simulink model "Induction_electromagnetique"  (R2017b)
settings: Solver=VariableStepAuto  StartTime=0.0  StopTime=inf  FixedStep=1/5000  RelTol=1e-3
libraries: fl_lib x16, Library_SII x4, nesl_utility x4, peRmsMeasurement x2
settings Model: Creator=Cedrick  LastModifiedBy=Cedrick

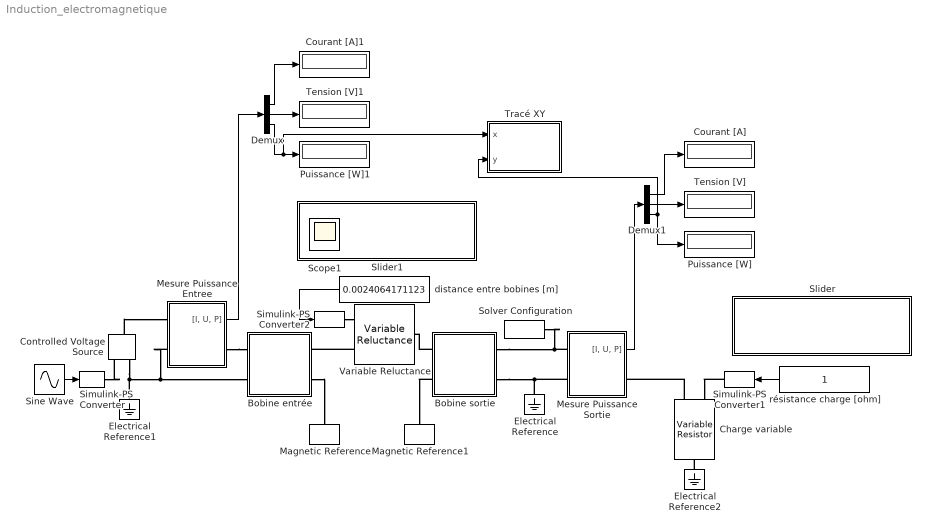
== system Induction_electromagnetique ==
  Bobine entrée : Subsystem  mask{N=30, s=1e-6, D=0.1, l=0.01}
      mask prompts: N "Nombre de tours"; s "Section du fil [m²]"; D "Diamètre de la bobine [m]"; l "Longueur de la bobine [m]"
      mask init:
      | % Perméabilité magnétique du vide
      | mu0 = pi*4e-7;
      | 
      | % Résistivité cuivre
      | rho = 1.7e-8; % Ohm.m
      mask DialogControl s Tooltip: Section du fil constituant la bobine
  Bobine sortie : Subsystem  mask{N=30, s=1e-6, D=0.1, l=0.01}
      mask prompts: N "Nombre de tours"; s "Section du fil [m²]"; D "Diamètre de la bobine [m]"; l "Longueur de la bobine [m]"
      mask init:
      | % Perméabilité magnétique du vide
      | mu0 = pi*4e-7;
      | 
      | % Résistivité cuivre
      | rho = 1.7e-8; % Ohm.m
      mask DialogControl s Tooltip: Section du fil constituant la bobine
  Charge variable : fl_lib/Electrical/Electrical Elements/Variable Resistor  Rmin=1 Ohm  i_specify=off  i_priority=None  i=0 A  i_nominal_specify=off  i_nominal_unit=A  i_nominal_value=1  v_specify=off  v_priority=None  v=0 V  v_nominal_specify=off  v_nominal_unit=V  v_nominal_value=1
  Controlled Voltage Source : fl_lib/Electrical/Electrical Sources/Controlled Voltage Source
  Courant [A] : Display
  Courant [A]1 : Display
  Demux : Demux  Outputs=3
  Demux1 : Demux  Outputs=3
  Electrical Reference : fl_lib/Electrical/Electrical Elements/Electrical Reference
  Electrical Reference1 : fl_lib/Electrical/Electrical Elements/Electrical Reference
  Electrical Reference2 : fl_lib/Electrical/Electrical Elements/Electrical Reference
  Magnetic Reference : fl_lib/Magnetic/Magnetic Elements/Magnetic Reference
      settings: SourceProductName=Simscape  SourceProductBaseCode=SS
  Magnetic Reference1 : fl_lib/Magnetic/Magnetic Elements/Magnetic Reference
      settings: SourceProductName=Simscape  SourceProductBaseCode=SS
  Mesure Puissance Entree : Subsystem  mask(Mesure de puissance Electrique RMS){ff=50}
      mask prompts: ff "Fréquence fondamentale [Hz]"
      mask help:
      | Mesure le courant, la tension et la puissance RMS sur un circuit.
      | Retourne les valeurs sous forme d'un vecteur [I, U, P]
      mask init:
      | fs = get_param(bdroot, 'FixedStep');
      | 
      | % Longueur de la fenêtre de mesure RMS
      | lw = int32(ff*fs)
      mask Display: disp('RMS')
  Mesure Puissance Sortie : Subsystem  mask(Mesure de puissance Electrique RMS){ff=50}
      mask prompts: ff "Fréquence fondamentale [Hz]"
      mask help:
      | Mesure le courant, la tension et la puissance RMS sur un circuit.
      | Retourne les valeurs sous forme d'un vecteur [I, U, P]
      mask init:
      | fs = get_param(bdroot, 'FixedStep');
      | 
      | % Longueur de la fenêtre de mesure RMS
      | lw = int32(ff*fs)
      mask Display: disp('RMS')
  Puissance [W] : Display
  Puissance [W]1 : Display
  Simulink-PS Converter : nesl_utility/Simulink-PS Converter  PhysicalDomain=network_engine_domain  SubClassName=ps_input  LeftPortType=input  RightPortType=output  PseudoPeriodic=off  Frequencies=[]  NoiseDistribution=none  NoiseParameters=[]  Unit=1  AffineConversion=off  FilteringAndDerivatives=provide  SimscapeFilterOrder=1  InputFilterTimeConstant=0.001  UdotUserProvided=0
  Simulink-PS Converter1 : nesl_utility/Simulink-PS Converter  PhysicalDomain=network_engine_domain  SubClassName=ps_input  LeftPortType=input  RightPortType=output  PseudoPeriodic=off  Frequencies=[]  NoiseDistribution=none  NoiseParameters=[]  Unit=1  AffineConversion=off  FilteringAndDerivatives=provide  SimscapeFilterOrder=1  InputFilterTimeConstant=0.001  UdotUserProvided=0
  Simulink-PS Converter2 : nesl_utility/Simulink-PS Converter  PhysicalDomain=network_engine_domain  SubClassName=ps_input  LeftPortType=input  RightPortType=output  PseudoPeriodic=off  Frequencies=[]  NoiseDistribution=none  NoiseParameters=[]  Unit=1  AffineConversion=off  FilteringAndDerivatives=provide  SimscapeFilterOrder=1  InputFilterTimeConstant=0.001  UdotUserProvided=0
  Sine Wave : Sin  Amplitude=5  Frequency=50*2*pi  SampleTime=0
  Slider : Subsystem  DialogController=hmiCreateDDGDialog  IsWebBlock=on  mask(MWDashboardBlock){webBlockId=574ab3c5-b9e4-429a-9142-107109e8eed0, webBlockType=slider, ShowInLibBrowser=on, ShowInitialText=on, HMISrcModelName=Induction}
      mask prompts: webBlockId "WebBlock Id"; webBlockType "WebBlock Type"; HMISrcModelName "Source Model"
      mask help: SimulinkHMI:dialogs:SliderDialogDesc
      mask Help: helpview([docroot '/mapfiles/simulink.map'], 'hmi_slider')
      mask Display:
      | if strcmp(get_param(bdroot(gcb),'BlockDiagramType'), 'library')
      |     image([(matlabroot) '/toolbox/simulink/hmi/icons/Slider.png']);
      | end
  Slider1 : Subsystem  DialogController=hmiCreateDDGDialog  IsWebBlock=on  mask(MWDashboardBlock){webBlockId=ceebdebb-3da2-42cb-9bc8-324251df0c3a, webBlockType=slider, ShowInLibBrowser=on, ShowInitialText=on, HMISrcModelName=Induction}
      mask prompts: webBlockId "WebBlock Id"; webBlockType "WebBlock Type"; HMISrcModelName "Source Model"
      mask help: SimulinkHMI:dialogs:SliderDialogDesc
      mask Help: helpview([docroot '/mapfiles/simulink.map'], 'hmi_slider')
      mask Display:
      | if strcmp(get_param(bdroot(gcb),'BlockDiagramType'), 'library')
      |     image([(matlabroot) '/toolbox/simulink/hmi/icons/Slider.png']);
      | end
  Solver Configuration : nesl_utility/Solver Configuration  PhysicalDomain=network_engine_domain  SubClassName=solver  LeftPortType=input  RightPortType=generic  Accelerate=off  Tones=[]  Harmonics=[]  SimulateNoise=off  Profile=off  UseLocalSampling=off  EnableSwitchedLinearOptims=on  FrequencyDomain=off  UseCCode=off  RelTol=0.001  AbsTol=1e-06  MinStep=1e-09  ToWorkspace=off  RevertToSquareIcSolve=off  NumHomotopyIterations=100  PhasorMode=off  PhasorModeNumHarmonics=1  DoDC=off  ResidualTolerance=1e-09  UseLocalSolver=off  LocalSolverChoice=NE_BACKWARD_EULER_ADVANCER  LocalSolverSampleTime=0.001  DoFixedCost=off  MaxNonlinIter=3  MaxModeIter=2  LinearAlgebra=Sparse  DelaysMemoryBudget=1024  AutomaticFiltering=on  FilteringTimeConstant=0.001
  Tension [V] : Display
  Tension [V]1 : Display
  Tracé XY : MATLAB Function  TreatAsAtomicUnit=on  SystemSampleTime=10
  Variable Reluctance : fl_lib/Magnetic/Magnetic Elements/Variable Reluctance  Xmin=0 m  CSA=pi*0.1^2/4 m^2  mur=1  phi_specify=off  phi_priority=None  phi=0 Wb  phi_nominal_specify=off  phi_nominal_unit=Wb  phi_nominal_value=1  mmf_specify=off  mmf_priority=None  mmf=0 A  mmf_nominal_specify=off  mmf_nominal_unit=A  mmf_nominal_value=1
      settings: SourceProductName=Simscape  SourceProductBaseCode=SS
  distance entre bobines [m] : Constant  Value=0.0024064171123
  résistance charge [ohm] : Constant
  Scope1 : Scope
  wires:
  Sine Wave/1 -> Simulink-PS Converter/1
  résistance charge [ohm]/1 -> Simulink-PS Converter1/1
  Demux1/1 -> Courant [A]/1
  Demux1/2 -> Tension [V]/1
  Demux1/3 -> Puissance [W]/1, Tracé XY/2(y)
  Demux/1 -> Courant [A]1/1
  Demux/2 -> Tension [V]1/1
  distance entre bobines [m]/1 -> Simulink-PS Converter2/1
  Demux/3 -> Tracé XY/1(x), Puissance [W]1/1
  Mesure Puissance Entree/1("[I, U, P]") -> Demux/1
  Mesure Puissance Sortie/1("[I, U, P]") -> Demux1/1
  connections:
  Bobine sortie/RConn1 -- Variable Reluctance/RConn1
  Solver Configuration/RConn1 -- Bobine sortie/LConn1 -- Mesure Puissance Sortie/LConn1
  Electrical Reference/LConn1 -- Bobine sortie/LConn2 -- Mesure Puissance Sortie/LConn2
  Controlled Voltage Source/RConn2 -- Electrical Reference1/LConn1 -- Mesure Puissance Entree/LConn2 -- Bobine entrée/LConn2
  Simulink-PS Converter/RConn1 -- Controlled Voltage Source/RConn1
  Variable Reluctance/LConn1 -- Bobine entrée/RConn1
  Simulink-PS Converter1/RConn1 -- Charge variable/LConn1
  Charge variable/LConn2 -- Mesure Puissance Sortie/RConn1
  Electrical Reference2/LConn1 -- Charge variable/RConn1
  Controlled Voltage Source/LConn1 -- Mesure Puissance Entree/LConn1
  Bobine sortie/RConn2 -- Magnetic Reference1/LConn1
  Bobine entrée/RConn2 -- Magnetic Reference/LConn1
  Mesure Puissance Entree/RConn1 -- Bobine entrée/LConn1
  Simulink-PS Converter2/RConn1 -- Variable Reluctance/LConn2

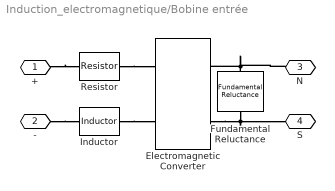
== system Induction_electromagnetique/Bobine entrée ==
  Electromagnetic Converter : fl_lib/Magnetic/Magnetic Elements/Electromagnetic Converter  Nw=N  i_specify=off  i_priority=None  i=0 A  i_nominal_specify=off  i_nominal_unit=A  i_nominal_value=1  v_specify=off  v_priority=None  v=0 V  v_nominal_specify=off  v_nominal_unit=V  v_nominal_value=1  mmf_specify=off  mmf_priority=None  mmf=0 A  mmf_nominal_specify=off  mmf_nominal_unit=A  mmf_nominal_value=1  phi_specify=off  phi_priority=High  phi=0 Wb  phi_nominal_specify=off  phi_nominal_unit=Wb  phi_nominal_value=1
      settings: SourceProductName=Simscape  SourceProductBaseCode=SS
  Fundamental Reluctance : fl_lib/Magnetic/Magnetic Elements/Fundamental Reluctance  R=4*l/(mu0*pi*D^2) 1/H  phi_specify=off  phi_priority=None  phi=0 Wb  phi_nominal_specify=off  phi_nominal_unit=Wb  phi_nominal_value=1  mmf_specify=off  mmf_priority=None  mmf=0 A  mmf_nominal_specify=off  mmf_nominal_unit=A  mmf_nominal_value=1
      settings: SourceProductName=Simscape  SourceProductBaseCode=SS
  Inductor : fl_lib/Electrical/Electrical Elements/Inductor  l=mu0*pi*D^2/4*N^2/l H  r=0 Ohm  g=1e-20 1/Ohm  i_specify=off  i_priority=None  i=0 A  i_nominal_specify=off  i_nominal_unit=A  i_nominal_value=1  v_specify=off  v_priority=None  v=0 V  v_nominal_specify=off  v_nominal_unit=V  v_nominal_value=1  i_L_specify=off  i_L_priority=High  i_L=0 A  i_L_nominal_specify=off  i_L_nominal_unit=A  i_L_nominal_value=1
  Resistor : fl_lib/Electrical/Electrical Elements/Resistor  R=rho*pi*D*N/s Ohm  i_specify=off  i_priority=None  i=0 A  i_nominal_specify=off  i_nominal_unit=A  i_nominal_value=1  v_specify=off  v_priority=None  v=0 V  v_nominal_specify=off  v_nominal_unit=V  v_nominal_value=1
  + : PMIOPort  Port=1  Side=Left
  - : PMIOPort  Port=2  Side=Left
  N : PMIOPort  Port=3  Side=Right
  S : PMIOPort  Port=4  Side=Right
  connections:
  Fundamental Reluctance/LConn1 -- Electromagnetic Converter/RConn1 -- N/RConn1
  Resistor/RConn1 -- Electromagnetic Converter/LConn1
  Electromagnetic Converter/RConn2 -- Fundamental Reluctance/RConn1 -- S/RConn1
  Inductor/RConn1 -- Electromagnetic Converter/LConn2
  +/RConn1 -- Resistor/LConn1
  -/RConn1 -- Inductor/LConn1

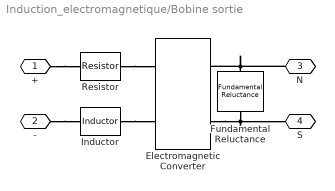
== system Induction_electromagnetique/Bobine sortie ==
  Electromagnetic Converter : fl_lib/Magnetic/Magnetic Elements/Electromagnetic Converter  Nw=N  i_specify=off  i_priority=None  i=0 A  i_nominal_specify=off  i_nominal_unit=A  i_nominal_value=1  v_specify=off  v_priority=None  v=0 V  v_nominal_specify=off  v_nominal_unit=V  v_nominal_value=1  mmf_specify=off  mmf_priority=None  mmf=0 A  mmf_nominal_specify=off  mmf_nominal_unit=A  mmf_nominal_value=1  phi_specify=off  phi_priority=High  phi=0 Wb  phi_nominal_specify=off  phi_nominal_unit=Wb  phi_nominal_value=1
      settings: SourceProductName=Simscape  SourceProductBaseCode=SS
  Fundamental Reluctance : fl_lib/Magnetic/Magnetic Elements/Fundamental Reluctance  R=4*l/(mu0*pi*D^2) 1/H  phi_specify=off  phi_priority=None  phi=0 Wb  phi_nominal_specify=off  phi_nominal_unit=Wb  phi_nominal_value=1  mmf_specify=off  mmf_priority=None  mmf=0 A  mmf_nominal_specify=off  mmf_nominal_unit=A  mmf_nominal_value=1
      settings: SourceProductName=Simscape  SourceProductBaseCode=SS
  Inductor : fl_lib/Electrical/Electrical Elements/Inductor  l=mu0*pi*D^2/4*N^2/l H  r=0 Ohm  g=1e-20 1/Ohm  i_specify=off  i_priority=None  i=0 A  i_nominal_specify=off  i_nominal_unit=A  i_nominal_value=1  v_specify=off  v_priority=None  v=0 V  v_nominal_specify=off  v_nominal_unit=V  v_nominal_value=1  i_L_specify=off  i_L_priority=High  i_L=0 A  i_L_nominal_specify=off  i_L_nominal_unit=A  i_L_nominal_value=1
  Resistor : fl_lib/Electrical/Electrical Elements/Resistor  R=rho*pi*D*N/s Ohm  i_specify=off  i_priority=None  i=0 A  i_nominal_specify=off  i_nominal_unit=A  i_nominal_value=1  v_specify=off  v_priority=None  v=0 V  v_nominal_specify=off  v_nominal_unit=V  v_nominal_value=1
  + : PMIOPort  Port=1  Side=Left
  - : PMIOPort  Port=2  Side=Left
  N : PMIOPort  Port=3  Side=Right
  S : PMIOPort  Port=4  Side=Right
  connections:
  N/RConn1 -- Fundamental Reluctance/LConn1 -- Electromagnetic Converter/RConn1
  Resistor/RConn1 -- Electromagnetic Converter/LConn1
  Electromagnetic Converter/RConn2 -- S/RConn1 -- Fundamental Reluctance/RConn1
  Inductor/RConn1 -- Electromagnetic Converter/LConn2
  +/RConn1 -- Resistor/LConn1
  -/RConn1 -- Inductor/LConn1

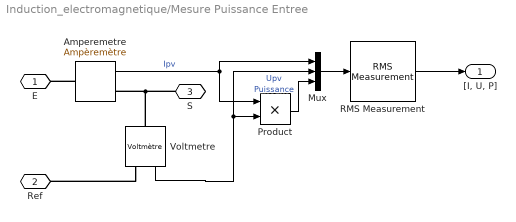
== system Induction_electromagnetique/Mesure Puissance Entree ==
  Amperemetre : Library_SII/Electronique/Ampèremètre
      settings: SourceProductName=SII
  Mux : Mux  Inputs=3
  Product : Product
  RMS Measurement : peRmsMeasurement/RMS Measurement  OverrideUsingVariant=Total  F=ff  SpecifyHarmonics=off  K=[0 1 2]  Ts=0
  Voltmetre : Library_SII/Electronique/Voltmètre
      settings: SourceProductName=SII
  E : PMIOPort  Port=1  Side=Left
  Ref : PMIOPort  Port=2  Side=Left
  S : PMIOPort  Port=3  Side=Right
  "[I, U, P]" : Outport
  wires:
  Amperemetre/1 -> Mux/1, Product/1  "Ipv"
  Voltmetre/1 -> Mux/2, Product/2  "Upv"
  Product/1 -> Mux/3  "Puissance"
  RMS Measurement/1 -> "[I, U, P]"/1
  Mux/1 -> RMS Measurement/1
  connections:
  Amperemetre/LConn1 -- E/RConn1
  Voltmetre/RConn1 -- Ref/RConn1
  Voltmetre/LConn1 -- S/RConn1 -- Amperemetre/RConn1

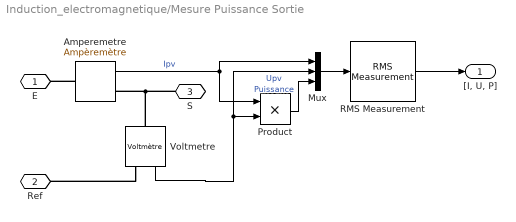
== system Induction_electromagnetique/Mesure Puissance Sortie ==
  Amperemetre : Library_SII/Electronique/Ampèremètre
      settings: SourceProductName=SII
  Mux : Mux  Inputs=3
  Product : Product
  RMS Measurement : peRmsMeasurement/RMS Measurement  OverrideUsingVariant=Total  F=ff  SpecifyHarmonics=off  K=[0 1 2]  Ts=0
  Voltmetre : Library_SII/Electronique/Voltmètre
      settings: SourceProductName=SII
  E : PMIOPort  Port=1  Side=Left
  Ref : PMIOPort  Port=2  Side=Left
  S : PMIOPort  Port=3  Side=Right
  "[I, U, P]" : Outport
  wires:
  Amperemetre/1 -> Mux/1, Product/1  "Ipv"
  Voltmetre/1 -> Mux/2, Product/2  "Upv"
  Product/1 -> Mux/3  "Puissance"
  RMS Measurement/1 -> "[I, U, P]"/1
  Mux/1 -> RMS Measurement/1
  connections:
  Amperemetre/LConn1 -- E/RConn1
  Voltmetre/RConn1 -- Ref/RConn1
  Voltmetre/LConn1 -- S/RConn1 -- Amperemetre/RConn1

== system Induction_electromagnetique/Slider ==

== system Induction_electromagnetique/Slider1 ==

== matlab function Induction_electromagnetique/Tracé XY ==
  data: x input; y input
function fcn(x, y)
coder.extrinsic('plot')
plot(x,y,'-o','Markersize',6,'MarkerFaceColor','g');
hold on;
set(gca,'XLim',[0 12],'Ylim',[0 6])
